simulink model "vipldwsRobot3"  (R2019a)
settings: Solver=FixedStepDiscrete  StartTime=0.0  StopTime=inf  RelTol=1e-3  EnableMultiTasking=on
model workspace (MATLAB code in the model file):
  | % Image size
  | imgSize = [240 360];
  | 
  | % Number of rows and columns in the image region to process.
  | numRows = floor(imgSize(1)/2);
  | numCols = imgSize(2);
  | 
  | % To handle different video sizes other than [240 360], scaling the Hough
  | % transform rho values by the below factor is required.
  | factor = sqrt(sum(imgSize.^2)) / sqrt(sum([240 360].^2));
  | 
  | %% parameters for the second lane
  | %approximately 35:45 (0-based index: 414:424)
  | startIdxRho_R = floor(factor * 414);
  | NumRhos_R = floor(factor * 11);
  | 
  | %approximately -90:-70 degrees (0-based index: 0:20)
  | startIdxTheta_R = 0;
  | NumThetas_R = 21;
  | neighborhood_R =  [min(7,NumRhos_R), min(7,NumThetas_R)];
  | 
  | %approximately 379:415 (0-based index: 0:35)
  | startIdxRho_L = floor(factor * 379);
  | NumRhos_L = floor(factor * 36);
  | 
  | %approximately 55:85 degrees (0-based index: 145: 175)
  | startIdxTheta_L = 145;
  | NumThetas_L = 21;
  | neighborhood_L =  [min(7,NumRhos_L), min(7,NumThetas_L)];
  | 
  | % Maximum number of lanes to find in the current frame.
  | expLaneNum = 2;
  | 
  | % Maximum number of lanes to store in the tracking repository.
  | maxLaneNum = 20;
  | 
  | % Angular resolution of Hough transform, i.e., the width of a theta bin is
  | % pi/angleNum.
  | angleNum = 180;
  | 
  | % Maximum allowable change of lane distance metric between two frames.
  | trackThreshold = 75;
  | 
  | % Minimum number of frames a lane must be detected to become a valid lane.
  | frameFound = 5;
  | 
  | % Maximum number of frames a lane can be missed without marking it invalid.
  | frameLost = 20;
  | 
  | % Size of the neighborhood around the maxima over which the Hough
  | % transforms values are suppressed. (Used in Find Local Maxima block)
  | neighborhood = [301, 81];
  | 
  | % Distance threshold for lane crossing warning; valid range is (0, 0.5).
  | thrWarn = 0.4;
  | 
  | % Weight (tweaking factor) of the angular difference for calculating the
  | % distance metric between two lanes. It is typically chosen to be close
  | % to the input image rows.
  | distanceMetricWeight = 200;
  | 
  | % Audio track used for lane cross warning.
  | load viprumbling.mat;
undefined symbols (not defined in the file or in its folder): gray, High, none, num_targets, Rec, SDTV, slselsubs, videoinput
libraries: simulink x19, visiontextngfix x8, robotlib x5, visiontransforms x4, dspmtrx3 x3, visionconversions x3, visionstatistics x3, dspsigops x2, dspindex x2, dspswit3 x2, dspstat3 x2, simulink_need_slupdate x2
(part 1 of 2)
settings Model: FPTRunName=Active  ExtModeAutoUpdateStatusClock=off  Creator=The MathWorks, Inc.  LastModifiedBy=ryoma
settings DataIOCC: LimitDataPoints=on  SaveFormat=Array  SaveOutput=off  SaveTime=off  ReturnWorkspaceOutputs=off
settings OptimizationCC: ExpressionDepthLimit=2147483647  LocalBlockOutputs=off  InitFltsAndDblsToZero=on  EfficientMapNaN2IntZero=off  LifeSpan=inf  BufferReusableBoundary=off
settings DebuggingCC: UnderspecifiedInitializationDetection=Classic  MergeDetectMultiDrivingBlocksExec=none  SignalResolutionControl=TryResolveAllWithWarning  SolverPrmCheckMsg=warning  InheritedTsInSrcMsg=none  MultiTaskDSMMsg=warning  SigSpecEnsureSampleTimeMsg=none  IntegerOverflowMsg=none  Int32ToFloatConvMsg=none  ParameterPrecisionLossMsg=none  FcnCallInpInsideContextMsg=warning  AllowSymbolicDim=off  UnknownTsInhSupMsg=none  StateNameClashWarn=warning  SFUnexpectedBacktrackingDiag=warning  SFNoUnconditionalDefaultTransitionDiag=warning  SFExecutionAtInitializationDiag=none  IntegerSaturationMsg=none  ArithmeticOperatorsInVariantConditions=warning
settings HardwareCC: ProdBitPerPointer=32  ProdBitPerSizeT=32  ProdBitPerPtrDiffT=32  ProdLargestAtomicFloat=None  ProdIntDivRoundTo=Undefined  ProdEndianess=Unspecified  ProdWordSize=32  ProdHWDeviceType=32-bit Generic  TargetBitPerPointer=64  TargetBitPerSizeT=64  TargetBitPerPtrDiffT=64  TargetLongLongMode=on  TargetIntDivRoundTo=Zero  TargetEndianess=LittleEndian  TargetWordSize=64  TargetHWDeviceType=Generic->MATLAB Host Computer  ProdEqTarget=off
settings ModelReferenceCC: PropagateSignalLabelsOutOfModel=off
settings SFSimCC: SimUseLocalCustomCode=off  SimParseCustomCode=off
settings RTWCC: RTWUseLocalCustomCode=off
settings CodeAppCC: StateflowObjectComments=on
settings GRTTargetCC: TargetFcnLib=ansi_tfl_tmw_new.mat  TargetLangStandard=C89/C90 (ANSI)  GeneratePreprocessorConditionals=Disable all  CombineOutputUpdateFcns=off  GRTInterface=on
settings ConfigComp: CovMetricSettings=dw  CovHtmlReporting=on  CovSaveCumulativeToWorkspaceVar=on  CovSaveSingleToWorkspaceVar=on  CovExternalEMLEnable=off

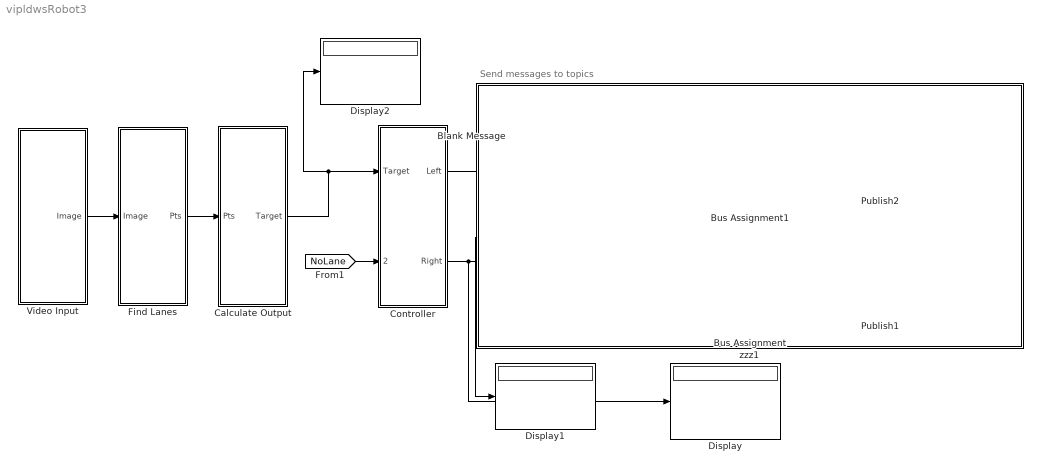
== system vipldwsRobot3 ==
  note: Send messages to topics
  Blank Message : robotlib/Blank Message  messageClass=Message  entityType=std_msgs/Int64  messageType=std_msgs/Int64  SampleTime=inf
      settings: SourceProductBaseCode=RO
  Bus Assignment : BusAssignment  AssignedSignals=Data
  Bus Assignment1 : BusAssignment  AssignedSignals=Data
  Calculate Output : Subsystem
  Controller : Subsystem
  Display : Display
  Display1 : Display
  Display2 : Display
  Find Lanes : Subsystem
  Publish1 : robotlib/Publish  topicSource=Select from ROS network  topic=/right_motor/cmd_vel  messageType=std_msgs/Int64  messageQueueLength=105
      settings: SourceProductBaseCode=RO
  Publish2 : robotlib/Publish  topicSource=Select from ROS network  topic=/left_motor/cmd_vel  messageType=std_msgs/Int64  messageQueueLength=105
      settings: SourceProductBaseCode=RO
  Video Input : Subsystem
  zzz1 : Subsystem  TreatAsAtomicUnit=on
      settings: OpenFcn=% no-op
      mask Display: disp('')
  wires:
  Video Input/1(Image) -> Find Lanes/1(Image)
  Find Lanes/1(Pts) -> Calculate Output/1(Pts)
  Bus Assignment1/1 -> Publish2/1
  Bus Assignment/1 -> Publish1/1
  Blank Message/1 -> Bus Assignment/1, Bus Assignment1/1
  Calculate Output/1(Target) -> Controller/1(Target), Display2/1
  [NoLane] -> Controller/2(No Lane)
  Controller/1(Left) -> Display1/1, Bus Assignment1/2
  Controller/2(Right) -> Bus Assignment/2, Display/1

== system vipldwsRobot3/Calculate Output ==
  Pts : Inport
  Add1 : Sum
  Constant : Constant  Value=160
  Convert 2-D to 1-D : dspsigattribs/Convert 2-D to 1-D
      settings: SourceProductName=DSP System Toolbox  SourceProductBaseCode=DS
  Demux1 : Demux  Outputs=8
  Display : Display
  Display1 : Display
  Gain : Gain  Gain=255/160
  Gain1 : Gain  Gain=.5
  Subtract : Sum  Inputs=+-
  Terminator{,1..5} (6 alike) : Terminator
  Target : Outport
  wires:
  Demux1/6 -> Add1/2, Display1/1  "right far x"
  Demux1/2 -> Display/1, Add1/1  "left far x"
  Pts/1 -> Convert 2-D to 1-D/1
  Convert 2-D to 1-D/1 -> Demux1/1
  Demux1/1 -> Terminator/1  "left far y"
  Demux1/3 -> Terminator1/1  "left close y"
  Demux1/4 -> Terminator2/1  "left close x"
  Demux1/5 -> Terminator3/1  "right far y"
  Demux1/7 -> Terminator4/1  "right close y"
  Demux1/8 -> Terminator5/1  "right close x"
  Constant/1 -> Subtract/2
  Add1/1 -> Gain1/1
  Gain1/1 -> Subtract/1
  Subtract/1 -> Gain/1
  Gain/1 -> Target/1

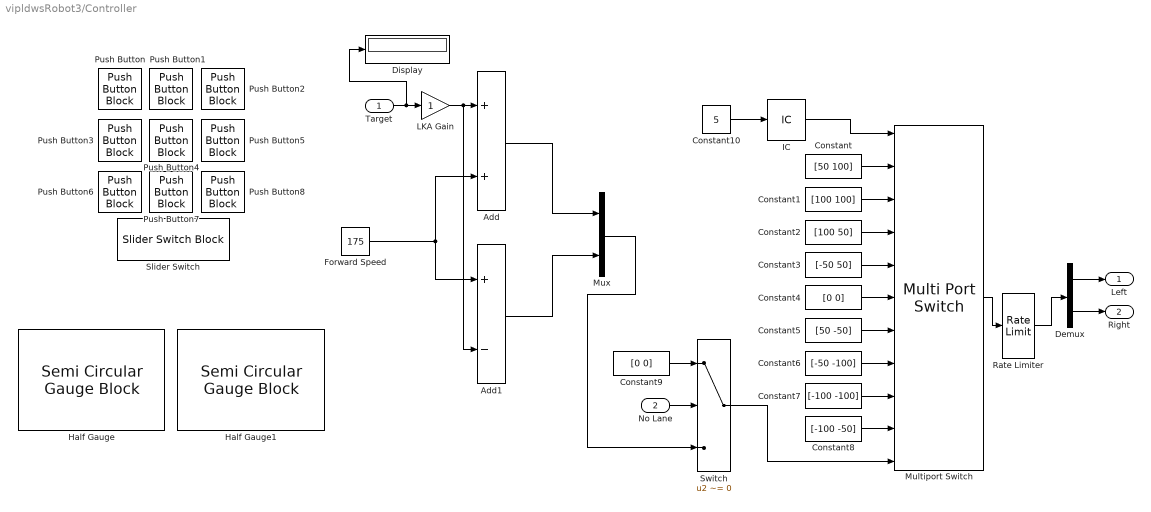
== system vipldwsRobot3/Controller ==
  Target : Inport
  No Lane : Inport  Port=2
  Add : Sum
  Add1 : Sum  Inputs=+-
  Constant : Constant  Value=[50 100]
  Constant1 : Constant  Value=[100 100]
  Constant10 : Constant  Value=5
  Constant2 : Constant  Value=[100 50]
  Constant3 : Constant  Value=[-50 50]
  Constant4 : Constant  Value=[0 0]
  Constant5 : Constant  Value=[50 -50]
  Constant6 : Constant  Value=[-50 -100]
  Constant7 : Constant  Value=[-100 -100]
  Constant8 : Constant  Value=[-100 -50]
  Constant9 : Constant  Value=[0 0]
  Demux : Demux  Outputs=2
  Display : Display
  Forward Speed : Constant  Value=175
  Half Gauge : SemiCircularGaugeBlock  ScaleMin=-255  ScaleMax=255
  Half Gauge1 : SemiCircularGaugeBlock  ScaleMin=-255  ScaleMax=255
  IC : InitialCondition  Value=5
  LKA Gain : Gain
  Multiport Switch : MultiPortSwitch  Inputs=10
  Mux : Mux  Inputs=2
  Push Button : PushButtonBlock  ButtonText=< /\
  Push Button1 : PushButtonBlock  ButtonText=/\  OnValue=2
  Push Button2 : PushButtonBlock  ButtonText=/\ >  OnValue=3
  Push Button3 : PushButtonBlock  ButtonText=<  OnValue=4
  Push Button4 : PushButtonBlock  ButtonText=0  OnValue=5
  Push Button5 : PushButtonBlock  ButtonText=>  OnValue=6
  Push Button6 : PushButtonBlock  ButtonText=< \/  OnValue=7
  Push Button7 : PushButtonBlock  ButtonText=\/  OnValue=8
  Push Button8 : PushButtonBlock  ButtonText=\/ >  OnValue=9
  Rate Limiter : RateLimiter  RisingSlewLimit=150  FallingSlewLimit=-150  SampleTimeMode=inherited
  Slider Switch : SliderSwitchBlock
      settings: Values={{'Off', 'On'}, [5 10]}
  Switch : Switch  Criteria=u2 ~= 0
  Left : Outport
  Right : Outport  Port=2
  wires:
  Forward Speed/1 -> Add1/1, Add/2
  Target/1 -> Display/1, LKA Gain/1
  LKA Gain/1 -> Add1/2, Add/1
  Add/1 -> Mux/1
  Add1/1 -> Mux/2
  No Lane/1 -> Switch/2
  Mux/1 -> Switch/3
  Rate Limiter/1 -> Demux/1
  Demux/1 -> Left/1
  Demux/2 -> Right/1
  Constant2/1 -> Multiport Switch/4
  Constant5/1 -> Multiport Switch/7
  Constant1/1 -> Multiport Switch/3
  Constant4/1 -> Multiport Switch/6
  Constant3/1 -> Multiport Switch/5
  Constant/1 -> Multiport Switch/2
  Constant7/1 -> Multiport Switch/9
  Constant8/1 -> Multiport Switch/10
  Multiport Switch/1 -> Rate Limiter/1
  Constant6/1 -> Multiport Switch/8
  Constant9/1 -> Switch/1
  Switch/1 -> Multiport Switch/11
  Constant10/1 -> IC/1
  IC/1 -> Multiport Switch/1

== system vipldwsRobot3/Find Lanes ==
  note: Lane Departure Warning System
  note: Double-click the Switch to specify
      | whether the demo highlights the lane
      | in front of the vehicle using a polygon or two lines.
  note: Copyright 2006-2011 The MathWorks, Inc.
  Image : Inport
  Departure Warning : Subsystem
  Draw Lines : Constant  Value=0  VectorParams1D=off  OutDataTypeStr=boolean
  Draw Polygon : Constant  VectorParams1D=off  OutDataTypeStr=boolean
  Info : vipmisc/Info  SystemSampleTime=-1
      settings: SourceProductName=Computer Vision Toolbox  SourceProductBaseCode=VP
  Input : Subsystem
  Lane Detection : Subsystem
  Lane Tracking : Subsystem
  Logical Operator : Logic  AllPortsSameDT=off  OutDataTypeStr=boolean
  Output : Subsystem
  Switch : ManualSwitch  CurrentSetting=0
  Pts : Outport
  wires:
  Departure Warning/4(Show3rdLane) -> Output/6(Show3rdLane)
  Input/4(YCbCrLow) -> [RefImg], Departure Warning/4(YCbCrLow)
  [R3rd] -> Output/8(R3rd)
  [RefImg] -> Output/10(RefImg)
  Draw Lines/1 -> Switch/1
  Image/1 -> Input/1("Image ")
  [L3rd] -> Output/9(L3rd)
  Input/2(EOF) -> Output/2(EOF), Lane Tracking/1(EOF)
  Input/3(ILow) -> Lane Detection/1(ILow), Departure Warning/3(ILow)
  Lane Tracking/1(Repository) -> Departure Warning/1(Repository)
  Departure Warning/6(TwoLanesFlag) -> Logical Operator/1, Output/11(TwoLanesFlag)
  Lane Detection/2(Enable) -> Lane Tracking/3(Enable)
  Departure Warning/3(Dis) -> Output/5(Dis)
  Lane Detection/1(Line) -> Lane Tracking/2(Line)
  Lane Tracking/2(Count) -> Departure Warning/2(Count)
  Departure Warning/5(ColorAndTypeIdx) -> Output/7(ColorAndTypeIdx)
  Departure Warning/1(Pts) -> Pts/1, Output/3(Pts)
  Departure Warning/2(Message) -> Output/4(Message)
  Draw Polygon/1 -> Switch/2
  Logical Operator/1 -> Output/12(ShowPolygon)
  Switch/1 -> Logical Operator/2
  Input/1(RGB) -> Output/1(RGB)
  Lane Detection/3(Right_3rdLane) -> [R3rd]
  Lane Detection/4(Left_3rdLane) -> [L3rd]

== system vipldwsRobot3/Video Input ==
  note: Receive messages sent to /usb_cam/image_raw topic
  After Blend : VideoViewer  FigPos=[46 541 418 304]
  Compositing1 : visiontextngfix/Compositing  operation=Blend  bFacSrc=Specify via dialog  bFactor=1  mFacSrc=Specify via dialog  mFactor=1  source=Specify via dialog  coordinates=[1 1]  roundingMode=Floor  overflowMode=off  firstCoeffSlope=2^-14  prodOutputMode=Binary point scaling  prodOutputWordLength=32  prodOutputFracLength=10  prodOutputSlope=2^-10  accumSlope=2^-10  outputSlope=2^-10
      settings: SourceProductName=Computer Vision Toolbox  SourceProductBaseCode=VP
  Constant : Constant  Value=[100 0 5 240; 220 0 5 240]  VectorParams1D=off  OutDataTypeStr=int32  SampleTime=1/30
  DrawShapes : visiontextngfix/Draw Shapes  shape=Rectangles  fill=on  lineWidth=1  fillClrSource=Specify via dialog  display=White  intensity=200  color=[255 255 255]  opacity=1  viewport=Entire image  antialiasing=off  inType=Obsolete  imagePorts=One multidimensional signal  roundingMode=Floor  overflowMode=off  memoryMode=Specify word length  memoryWordLength=16  prodOutputMode=Binary point scaling  prodOutputWordLength=32  prodOutputFracLength=14  prodOutputSlope=2^-14  accumSlope=2^-14  memoryFracLength=14
      settings: SourceProductName=Computer Vision Toolbox
  From Video Device : imaqlib/From Video Device  DeviceMenu=winvideo 1 (HD WebCam)  Device=winvideo 1 (HD WebCam)  ObjConstructor=videoinput('winvideo', 1)  VideoFormatMenu=MJPG_640x480  VideoFormat=MJPG_640x480  VideoSource=input1  ROIPosition=[0 0 480 640]  EnableHWTrigger=off  TriggerConfiguration=none/none  SampleTime=1/30  OutputPortsMode=One multidimensional signal  DataType=single  CanDoHWTrigger=no  ReturnedColorSpace=rgb  BlockHandle=1351.0002  ROIWidth=640  ROIHeight=480  ROIColumn=0  ROIRow=0  EngXMLPath=C:\Program Files\MATLAB\R2019a\toolbox\imaq\imaq\private  DevXMLPath=C:\ProgramData\MATLAB\SupportPackages\R2019a\toolbox\imaq\supportpackages\genericvideo\adaptor\win64  EngLibPath=C:\Program Files\MATLAB\R2019a\toolbox\imaq\imaqblks\imaqmex\win64  ColorSpace=rgb  BayerSensorAlignment=grbg  ImaqMode=off
      settings: SourceProductName=Image Acquisition Toolbox
  Image From File : visionsources/Image From File  Tag=vipblks_nd  FileName=C:\Users\ryoma\Desktop\rosmotor\windows\1x1.png  Ts=1/30  imagePorts=One multidimensional signal  OutPortLabels=R|G|B  ImageDataType=Inherit from input image  sdImageDataType=uint(8)  Signed=on  WordLength=16  FractionLengthMode=User-defined  FractionLength=15
      settings: SourceProductName=Computer Vision Toolbox
  Read Image : robotlib/Read Image  MaximumImageSize=[480, 640]  ImageEncoding=rgb8  ShowAlphaOutput=off  ShowErrorCodeOutput=off  VariableSizeOutputs=off
      settings: SourceProductName=Robotics System Toolbox  SourceProductBaseCode=RO
  Resize : visiongeotforms/Resize  specify=Output size as a percentage of input size  rfactor=50  outCols=25  outRows=25  outRowsCols=[25 35]  interp_method=Bilinear  antialias=on  useROI=off  roiFlag=off  roundingMode=Nearest  overflowMode=on  prodOutputMode=Binary point scaling  prodOutputWordLength=32  prodOutputFracLength=10  prodOutputSlope=2^-10  accumSlope=2^-10  outputSlope=2^-10
      settings: SourceProductName=Computer Vision Toolbox  SourceProductBaseCode=VP
  Resize1 : visiongeotforms/Resize  specify=Output size as a percentage of input size  rfactor=50  outCols=25  outRows=25  outRowsCols=[25 35]  interp_method=Bilinear  antialias=on  useROI=off  roiFlag=off  roundingMode=Nearest  overflowMode=on  prodOutputMode=Binary point scaling  prodOutputWordLength=32  prodOutputFracLength=10  prodOutputSlope=2^-10  accumSlope=2^-10  outputSlope=2^-10
      settings: SourceProductName=Computer Vision Toolbox  SourceProductBaseCode=VP
  Sample and Hold : dspsigops/Sample and Hold  Commented=on  trig=Rising edge  initCond=0  latchinput=off
  Step : Step  SampleTime=1/30
  Subscribe1 : robotlib/Subscribe  topicSource=Select from ROS network  topic=/usb_cam/image_raw  messageType=sensor_msgs/Image  sampleTime=1/30  messageQueueLength=51
      settings: SourceProductBaseCode=RO
  Switch : Switch  Criteria=u2 > Threshold
  zzz2 : Subsystem  TreatAsAtomicUnit=on
      settings: OpenFcn=% no-op
      mask Display: disp('')
  Image : Outport
  wires:
  From Video Device/1 -> Resize/1
  Subscribe1/2 -> Read Image/1
  Subscribe1/1 -> Sample and Hold/Trigger
  Read Image/1 -> Resize1/1
  DrawShapes/1 -> Switch/3
  Constant/1 -> DrawShapes/2
  Step/1 -> Switch/2
  Resize1/1 -> Compositing1/2
  Compositing1/1 -> DrawShapes/1, Switch/1, After Blend/1
  Image From File/1 -> Compositing1/1
  Switch/1 -> Image/1

== system vipldwsRobot3/zzz1 ==

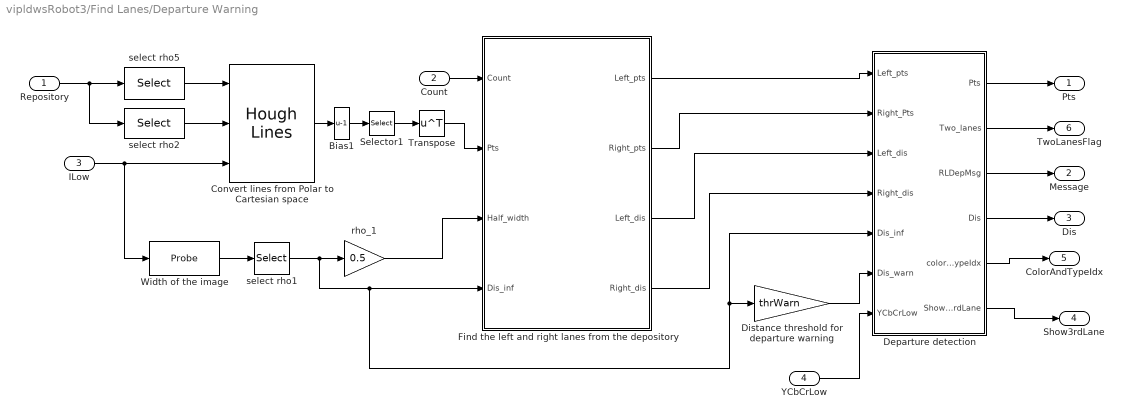
== system vipldwsRobot3/Find Lanes/Departure Warning ==
  Repository : Inport
  Count : Inport  Port=2
  ILow : Inport  Port=3
  YCbCrLow : Inport  Port=4
  Bias1 : Bias  Bias=-1
  Convert lines from Polar to Cartesian space : visiontransforms/Hough Lines  sineCompMethod=Trigonometric function  thetaRes=pi/180  roundingMode=Nearest  overflowMode=on  firstCoeffMode=Specify word length  firstCoeffWordLength=16  prodOutputMode=Binary point scaling  prodOutputWordLength=32  prodOutputFracLength=16  prodOutputSlope=2^-16  accumSlope=2^-16  firstCoeffFracLength=15
      settings: SourceProductName=Computer Vision Toolbox  SourceProductBaseCode=VP
  Departure detection : Subsystem
  Distance threshold for departure warning : Gain  Gain=thrWarn  OutDataTypeStr=Inherit: Same as input
  Find the left and right lanes from the depository : Subsystem  TreatAsAtomicUnit=on
  Selector1 : Selector  NumberOfDimensions=2  InputPortWidth=3  IndexOptions=Select all,Index vector (dialog)  Indices=[2 1],[2 1 4 3]  OutputSizes=1,1
  Transpose : Math  Operator=transpose  SaturateOnIntegerOverflow=on
  Width of the image : Probe  ProbeWidth=off  ProbeSampleTime=off  ProbeComplexSignal=off  ProbeSignalDimensions=on  ProbeDimensionsDataType=int32
  rho_1 : Gain  Gain=0.5  OutDataTypeStr=Inherit: Same as input
  select rho1 : Selector  InputPortWidth=2  IndexOptions=Index vector (dialog)  Indices=2  OutputSizes=1
  select rho2 : Selector  NumberOfDimensions=2  InputPortWidth=maxLaneNum  IndexOptions=Index vector (dialog),Select all  Indices=1,-1  OutputSizes=1
  select rho5 : Selector  NumberOfDimensions=2  InputPortWidth=maxLaneNum  IndexOptions=Index vector (dialog),Select all  Indices=2,-1  OutputSizes=1
  Pts : Outport
  Message : Outport  Port=2
  Dis : Outport  Port=3
  Show3rdLane : Outport  Port=4
  ColorAndTypeIdx : Outport  Port=5
  TwoLanesFlag : Outport  Port=6
  wires:
  select rho2/1 -> Convert lines from Polar to Cartesian space/2
  Count/1 -> Find the left and right lanes from the depository/1(Count)
  Repository/1 -> select rho5/1, select rho2/1
  ILow/1 -> Convert lines from Polar to Cartesian space/3, Width of the image/1
  select rho1/1 -> rho_1/1, Find the left and right lanes from the depository/4(Dis_inf), Distance threshold for departure warning/1, Departure detection/5(Dis_inf)
  Find the left and right lanes from the depository/2(Right_pts) -> Departure detection/2(Right_Pts)
  Find the left and right lanes from the depository/1(Left_pts) -> Departure detection/1(Left_pts)
  rho_1/1 -> Find the left and right lanes from the depository/3(Half_width)
  Width of the image/1 -> select rho1/1
  Find the left and right lanes from the depository/3(Left_dis) -> Departure detection/3(Left_dis)
  Find the left and right lanes from the depository/4(Right_dis) -> Departure detection/4(Right_dis)
  Distance threshold for departure warning/1 -> Departure detection/6(Dis_warn)
  Departure detection/1(Pts) -> Pts/1
  Departure detection/2(Two_lanes) -> TwoLanesFlag/1
  Departure detection/3(RLDepMsg) -> Message/1
  Departure detection/4(Dis) -> Dis/1
  select rho5/1 -> Convert lines from Polar to Cartesian space/1
  YCbCrLow/1 -> Departure detection/7(YCbCrLow)
  Departure detection/6(Show3rdLane) -> Show3rdLane/1
  Departure detection/5(colorAndTypeIdx) -> ColorAndTypeIdx/1
  Selector1/1 -> Transpose/1
  Convert lines from Polar to Cartesian space/1 -> Bias1/1
  Transpose/1 -> Find the left and right lanes from the depository/2(Pts)
  Bias1/1 -> Selector1/1

== system vipldwsRobot3/Find Lanes/Input ==
  note: For different video sizes, set imgSize appropriately in model
      | workspace and then press the "Reinitialize from Source" button.
  "Image " : Inport
  Clip image : dspmtrx3/Submatrix  RowSpan=Range of rows  RowStartMode=Index  RowStartIndex=numRows+1  RowEndMode=Last  RowEndIndex=1  ColSpan=All columns  ColStartMode=First  ColStartIndex=1  ColEndMode=Last  ColEndIndex=1
  Color Space Conversion : visionconversions/Color Space  Conversion  conversion=Obsolete  conversionActive=R'G'B' to intensity  wp_str=D65  rec=Rec. 601 (SDTV)  sys=1125/60/2:1  imagePorts=One multidimensional signal
  Color Space Conversion1 : visionconversions/Color Space  Conversion  conversion=Obsolete  conversionActive=R'G'B' to Y'CbCr  wp_str=D65  rec=Rec. 601 (SDTV)  sys=1125/60/2:1  imagePorts=One multidimensional signal
  From Multimedia File1 : dspvision/From Multimedia File  Commented=on  inputFilename=viplanedeparture.mp4  readRange=[1 Inf]  loop=on  numPlays=inf  outputStreams=Video only  videoDataType=single  audioDataType=int16  inheritSampleTime=off  userDefinedSampleTime=1/30  noAudioOutput=off  isIntensityVideo=off  fourcc=RGB  colorVideoFormat=One multidimensional signal  outputEOF=on  dataOrg=Column-major  audioFrameSize=1024  computeAudioFrameSize=off  outSamplingMode=Frame based
      settings: SourceProductName=DSP System Toolbox  SourceProductBaseCode=DS
  OR : Logic  Operator=OR  IconShape=distinctive  AllPortsSameDT=off  OutDataTypeStr=boolean
  Selector : Selector  NumberOfDimensions=3  InputPortWidth=3  IndexOptions=Index vector (dialog),Select all,Select all  Indices=(numRows+1):imgSize(1),1,2  OutputSizes=1,1,1
  RGB : Outport
  EOF : Outport  Port=2
  ILow : Outport  Port=3
  YCbCrLow : Outport  Port=4
  tag scope: NoLane=global
  wires:
  Color Space Conversion/1 -> Clip image/1
  Clip image/1 -> ILow/1
  Selector/1 -> Color Space Conversion1/1
  Color Space Conversion1/1 -> YCbCrLow/1
  "Image "/1 -> Selector/1, Color Space Conversion/1, RGB/1
  [Lane0R] -> OR/2
  [Lane0L] -> OR/1
  OR/1 -> EOF/1, [NoLane]

== system vipldwsRobot3/Find Lanes/Lane Detection ==
  ILow : Inport
  2-D FIR Filter : visionfilter/2-D FIR Filter  separable=off  filtSrc=Specify via dialog  filterMtrx=[-1 0 1]  verticalFilter=[4 0]  horizontalFilter=[4 0]  outSize=Same as input port I  padType=Replicate  padSrc=Specify via dialog  padVal=0  method=Correlation  firstCoeffMode=Specify word length  firstCoeffWordLength=16  firstCoeffFracLength=14  firstCoeffSignedness=Signed  firstCoeffLastDataTypeStr=fixdt(1,16)  outputSignedness=Auto  accumLastDataTypeStr=Inherit: Same as product output  prodOutputMode=Binary point scaling  prodOutputWordLength=32  prodOutputFracLength=10  prodOutputLastDataTypeStr=fixdt([],32,10)  roundingMode=Floor  overflowMode=on  firstCoeffDataTypeStr=fixdt(1,16)  firstCoeffMin=[]  firstCoeffMax=[]  prodOutputDataTypeStr=fixdt([],32,10)  accumDataTypeStr=Inherit: Same as product output  outputMin=[]  outputMax=[]
      settings: SourceProductName=Computer Vision Toolbox  SourceProductBaseCode=VP
  3rd lane: Right-Left : Subsystem
  Hough Transform : visiontransforms/Hough Transform  theta_res=pi/angleNum  rho_res=1  out_theta_rho=on  outdtmode=single  roundingMode=Nearest  overflowMode=on  firstCoeffMode=Binary point scaling  firstCoeffWordLength=16  firstCoeffFracLength=14  firstCoeffSlope=2^-14  secondCoeffMode=Binary point scaling  secondCoeffWordLength=32  secondCoeffFracLength=16  secondCoeffSlope=2^-16  prodOutputMode=Binary point scaling  prodOutputWordLength=32  prodOutputFracLength=20  prodOutputSlope=2^-20  accumMode=Binary point scaling  accumWordLength=32  accumFracLength=20  accumSlope=2^-20  outputMode=Binary point scaling  outputWordLength=16  outputFracLength=0  outputSlope=2^0  memoryMode=Binary point scaling  memoryWordLength=32  memoryFracLength=16  memorySlope=2^-16
      settings: SourceProductName=Computer Vision Toolbox  SourceProductBaseCode=VP
  Image thresholding : visionconversions/Autothreshold  operator=>  threshOut=off  effMetricOut=off  userDefinedRange=off  umin=0  umax=255  outOfRngOpt=Warn and saturate  scaleThreshold=off  scaleFactor=1  roundingMode=Floor  overflowMode=off  P1Mode=Specify word length  P1WordLength=32  P1FracLength=30  P1Slope=2^-30  A1Slope=2^-30  P2Mode=Specify word length  P2WordLength=32  P2FracLength=22  P2Slope=2^-22  A2Slope=2^-22  P3Mode=Specify word length  P3WordLength=32  P3FracLength=14  P3Slope=2^-14  A3Slope=2^-14  P4Mode=Binary point scaling  P4WordLength=32  P4FracLength=15  P4Slope=2^-15  A4Slope=2^-4  Q1Mode=Specify word length  Q1WordLength=32  Q1FracLength=16  Q1Slope=2^-16  EMMode=Specify word length  EMWordLength=16  EMFracLength=14  EMSlope=2^-14
      settings: SourceProductName=Computer Vision Toolbox  SourceProductBaseCode=VP
  Overwrite : Subsystem
  Peak detection : Subsystem
  Saturation : Saturate  UpperLimit=1  LowerLimit=0
  Line : Outport
  Enable : Outport  Port=2
  Right_3rdLane : Outport  Port=3
  Left_3rdLane : Outport  Port=4
  wires:
  Overwrite/1(Out) -> Peak detection/1(Hough)
  3rd lane: Right-Left/2(LeftPts) -> Left_3rdLane/1
  3rd lane: Right-Left/1(RightPts) -> Right_3rdLane/1
  Peak detection/2(Enable) -> Enable/1
  Peak detection/1(Line) -> Line/1
  Hough Transform/3 -> Peak detection/3(Rho_list), 3rd lane: Right-Left/3(rho_list)
  Hough Transform/2 -> Peak detection/2(Theta_list), 3rd lane: Right-Left/2(th_list)
  Hough Transform/1 -> Overwrite/1(In), 3rd lane: Right-Left/1(H)
  Saturation/1 -> Image thresholding/1
  2-D FIR Filter/1 -> Saturation/1
  Image thresholding/1 -> Hough Transform/1
  ILow/1 -> 2-D FIR Filter/1, 3rd lane: Right-Left/4(Ref I)

== system vipldwsRobot3/Find Lanes/Lane Tracking ==
  EOF : Inport
  Line : Inport  Port=2
  Enable : Inport  Port=3
  Kalman Filter : dspadpt3/Kalman Filter  num_targets=maxLaneNum  sourceEnable=Specify via input port <Enable>  isReset=on  X=zeros([4, 1])  P=100*eye(4)  A=[1 0 1 0;0 1 0 1; 0 0 1 0; 0 0 0 1]  sourceMeasure=Specify via Dialog  H=[1 0 0 0; 0 1 0 0]  Q=0.05*eye(4)  R=1*eye(2)  isOutputEstMeasure=on  isOutputEstState=off  isOutputEstError=off  isOutputPrdMeasure=on  isOutputPrdState=off  isOutputPrdError=off
      settings: SourceProductName=DSP System Toolbox  SourceProductBaseCode=DS
  Matching : Subsystem
  Only update the lines which Kalman filter has been trained for enough time : simulink/Logic and Bit Operations/Compare To Constant  relop=>=  const=frameFound  OutDataTypeStr=boolean  ZeroCross=off
  Unit Delay Resettable : simulink_need_slupdate/Unit Delay Resettable  vinit=0  tsamp=-1
      settings: SourceProductName=Simulink  SourceProductBaseCode=SL
  Unit Delay Resettable1 : simulink_need_slupdate/Unit Delay Resettable  vinit=zeros(2,maxLaneNum)  tsamp=-1
      settings: SourceProductName=Simulink  SourceProductBaseCode=SL
  Update : Subsystem  TreatAsAtomicUnit=on
  Repository : Outport
  Count : Outport  Port=2
  wires:
  Matching/2(Count) -> Unit Delay Resettable/1, Only update the lines which Kalman filter has been trained for enough time/1, Count/1, Kalman Filter/2
  Only update the lines which Kalman filter has been trained for enough time/1 -> Update/3(Update)
  Unit Delay Resettable/1 -> Matching/4(Count_ref)
  Unit Delay Resettable1/1 -> Matching/3(Rep_ref)
  Line/1 -> Matching/1(Line)
  Enable/1 -> Matching/2(Enable)
  Matching/1(Repository) -> Update/1(Old), Kalman Filter/1
  Update/1(Out) -> Unit Delay Resettable1/1
  Kalman Filter/2 -> Update/2(New)
  Kalman Filter/1 -> Repository/1
  EOF/1 -> Unit Delay Resettable1/2, Unit Delay Resettable/2

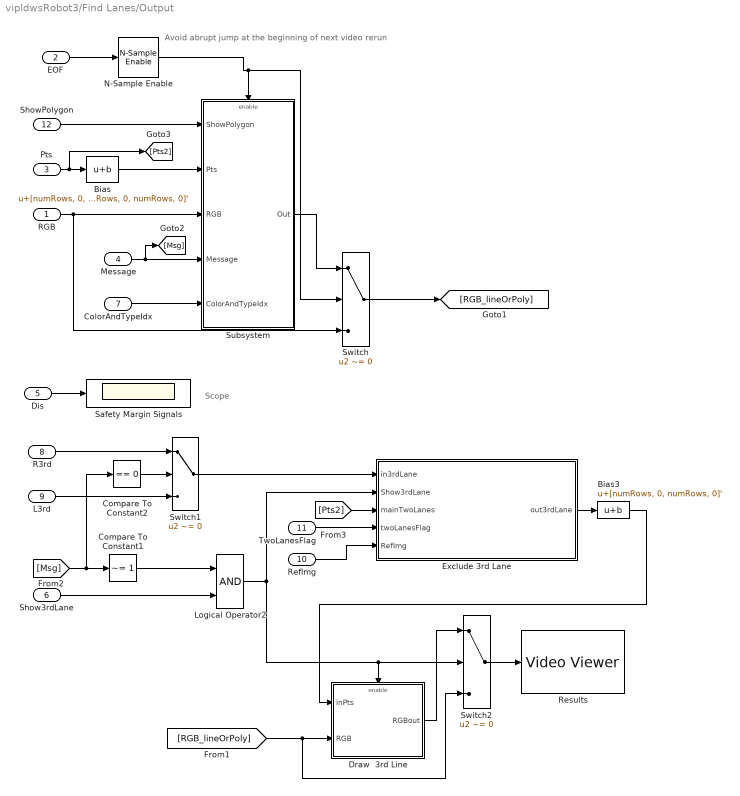
== system vipldwsRobot3/Find Lanes/Output ==
  note: Scope
  note: Avoid abrupt jump at the beginning of next video rerun
  RGB : Inport
  EOF : Inport  Port=2
  Pts : Inport  Port=3
  Message : Inport  Port=4
  Dis : Inport  Port=5
  Show3rdLane : Inport  Port=6
  ColorAndTypeIdx : Inport  Port=7
  R3rd : Inport  Port=8
  L3rd : Inport  Port=9
  RefImg : Inport  Port=10
  TwoLanesFlag : Inport  Port=11
  ShowPolygon : Inport  Port=12
  Bias : Bias  Bias=[numRows, 0, numRows, 0; numRows, 0, numRows, 0]'
  Bias3 : Bias  Bias=[numRows, 0, numRows, 0]'
  Compare To Constant1 : simulink/Logic and Bit Operations/Compare To Constant  relop=~=  const=1  OutDataTypeStr=boolean  ZeroCross=off
  Compare To Constant2 : simulink/Logic and Bit Operations/Compare To Constant  relop===  const=0  OutDataTypeStr=boolean  ZeroCross=off
  Draw  3rd Line : Subsystem  TreatAsAtomicUnit=on
  Exclude 3rd Lane : MATLAB Function  TreatAsAtomicUnit=on
  Logical Operator2 : Logic  AllPortsSameDT=off  OutDataTypeStr=boolean
  N-Sample Enable : dspswit3/N-Sample Enable  N=8  ActiveLevel=High (1)  reset=on  TriggerType=Non-zero sample  Ts=1  DataType=Logical
      settings: SourceProductName=DSP System Toolbox  SourceProductBaseCode=DS
  Results : VideoViewer  colormapValue=gray(256)  FigPos=[842 424 491 266]
  Safety Margin Signals : Scope
  Subsystem : Subsystem
  Switch : Switch  Criteria=u2 ~= 0
  Switch1 : Switch  Criteria=u2 ~= 0  ZeroCross=off
  Switch2 : Switch  Criteria=u2 ~= 0
  wires:
  Pts/1 -> Bias/1, [Pts2]
  Message/1 -> Subsystem/4(Message), [Msg]
  Dis/1 -> Safety Margin Signals/1
  Bias/1 -> Subsystem/2(Pts)
  ColorAndTypeIdx/1 -> Subsystem/5(ColorAndTypeIdx)
  Show3rdLane/1 -> Logical Operator2/2
  [RGB_lineOrPoly] -> Draw  3rd Line/2(RGB), Switch2/3
  [Msg] -> Compare To Constant1/1, Compare To Constant2/1
  Compare To Constant1/1 -> Logical Operator2/1
  Logical Operator2/1 -> Exclude 3rd Lane/2(Show3rdLane), Draw  3rd Line/Enable, Switch2/2
  Compare To Constant2/1 -> Switch1/2
  Switch1/1 -> Exclude 3rd Lane/1(in3rdLane)
  Draw  3rd Line/1(RGBout) -> Switch2/1
  Switch2/1 -> Results/1
  [Pts2] -> Exclude 3rd Lane/3(mainTwoLanes)
  TwoLanesFlag/1 -> Exclude 3rd Lane/4(twoLanesFlag)
  RefImg/1 -> Exclude 3rd Lane/5(RefImg)
  Exclude 3rd Lane/1(out3rdLane) -> Bias3/1
  R3rd/1 -> Switch1/1
  L3rd/1 -> Switch1/3
  ShowPolygon/1 -> Subsystem/1(ShowPolygon)
  RGB/1 -> Subsystem/3(RGB), Switch/3
  N-Sample Enable/1 -> Switch/2, Subsystem/Enable
  EOF/1 -> N-Sample Enable/1
  Bias3/1 -> Draw  3rd Line/1(inPts)
  Switch/1 -> [RGB_lineOrPoly]
  Subsystem/1(Out) -> Switch/1

== system vipldwsRobot3/Video Input/zzz2 ==

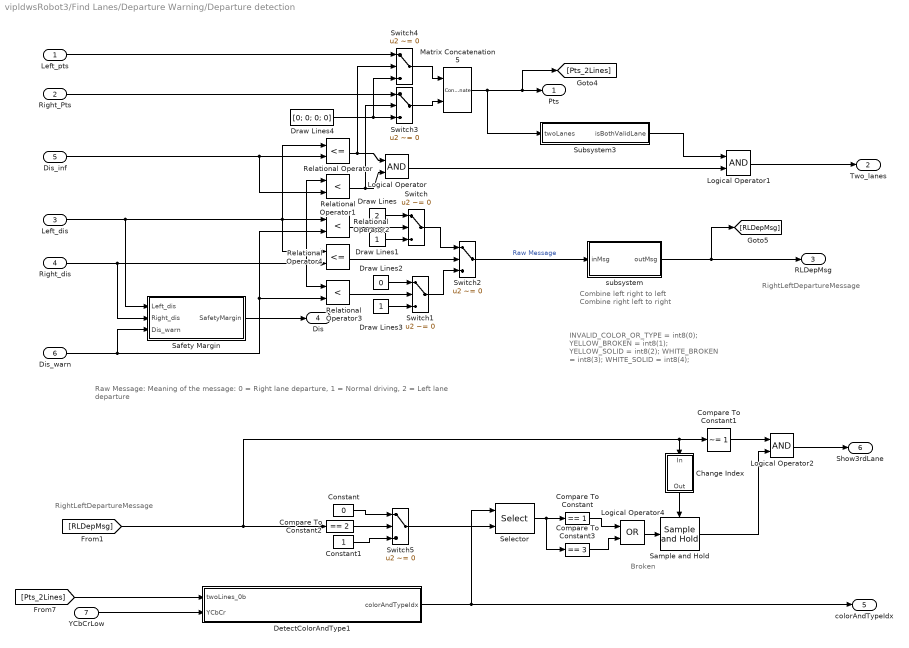
== system vipldwsRobot3/Find Lanes/Departure Warning/Departure detection ==
  note: Raw Message:
      | Meaning of the message: 0 = Right lane departure, 1 = Normal driving, 2 = Left lane departure
  note: RightLeftDepartureMessage
  note: INVALID_COLOR_OR_TYPE = int8(0);
      | YELLOW_BROKEN  = int8(1);
      | YELLOW_SOLID      = int8(2);
      | WHITE_BROKEN     = int8(3);
      | WHITE_SOLID         = int8(4);
  note: Broken
  note: RightLeftDepartureMessage
  note: Combine left right to left
      | Combine right left to right
  Left_pts : Inport
  Right_Pts : Inport  Port=2
  Left_dis : Inport  Port=3
  Right_dis : Inport  Port=4
  Dis_inf : Inport  Port=5
  Dis_warn : Inport  Port=6
  YCbCrLow : Inport  Port=7
  Change Index : Subsystem
  Compare To Constant : simulink/Logic and Bit Operations/Compare To Constant  relop===  const=1  OutDataTypeStr=boolean  ZeroCross=off
  Compare To Constant1 : simulink/Logic and Bit Operations/Compare To Constant  relop=~=  const=1  OutDataTypeStr=boolean  ZeroCross=off
  Compare To Constant2 : simulink/Logic and Bit Operations/Compare To Constant  relop===  const=2  OutDataTypeStr=boolean  ZeroCross=off
  Compare To Constant3 : simulink/Logic and Bit Operations/Compare To Constant  relop===  const=3  OutDataTypeStr=boolean  ZeroCross=off
  Constant : Constant  Value=0  VectorParams1D=off  OutDataTypeStr=int8
  Constant1 : Constant  VectorParams1D=off  OutDataTypeStr=int8
  DetectColorAndType1 : MATLAB Function  TreatAsAtomicUnit=on
  Draw Lines : Constant  Value=2  VectorParams1D=off  OutDataTypeStr=int8  SampleTime=-1
  Draw Lines1 : Constant  VectorParams1D=off  OutDataTypeStr=int8  SampleTime=-1
  Draw Lines2 : Constant  Value=0  VectorParams1D=off  OutDataTypeStr=int8  SampleTime=-1
  Draw Lines3 : Constant  VectorParams1D=off  OutDataTypeStr=int8  SampleTime=-1
  Draw Lines4 : Constant  Value=[0; 0; 0; 0]  VectorParams1D=off  OutDataTypeStr=int32  SampleTime=-1
  Logical Operator : Logic  AllPortsSameDT=off  OutDataTypeStr=boolean
  Logical Operator1 : Logic  AllPortsSameDT=off  OutDataTypeStr=boolean
  Logical Operator2 : Logic  AllPortsSameDT=off  OutDataTypeStr=boolean
  Logical Operator4 : Logic  Operator=OR  AllPortsSameDT=off  OutDataTypeStr=boolean
  Matrix Concatenation5 : Concatenate  Mode=Multidimensional array  ConcatenateDimension=2
  Relational Operator : RelationalOperator  Operator=<=  OutDataTypeStr=boolean  ZeroCross=off  RndMeth=Nearest
  Relational Operator1 : RelationalOperator  Operator=<  OutDataTypeStr=boolean  ZeroCross=off  RndMeth=Nearest
  Relational Operator2 : RelationalOperator  Operator=<  OutDataTypeStr=boolean  ZeroCross=off  RndMeth=Nearest
  Relational Operator3 : RelationalOperator  Operator=<  OutDataTypeStr=boolean  ZeroCross=off  RndMeth=Nearest
  Relational Operator4 : RelationalOperator  Operator=<=  OutDataTypeStr=boolean  ZeroCross=off  RndMeth=Nearest
  Safety Margin : Subsystem
  Sample and Hold : dspsigops/Sample and Hold  trig=Either edge  initCond=0  latchinput=off
  Selector : Selector  IndexMode=Zero-based  InputPortWidth=2  IndexOptions=Index vector (port)  Indices=[1 3]  OutputSizes=1
  Subsystem3 : Subsystem
  Switch : Switch  Criteria=u2 ~= 0
  Switch1 : Switch  Criteria=u2 ~= 0
  Switch2 : Switch  Criteria=u2 ~= 0
  Switch3 : Switch  Criteria=u2 ~= 0  ZeroCross=off
  Switch4 : Switch  Criteria=u2 ~= 0  ZeroCross=off
  Switch5 : Switch  Criteria=u2 ~= 0  ZeroCross=off
  subsystem : Subsystem
  Pts : Outport
  Two_lanes : Outport  Port=2
  RLDepMsg : Outport  Port=3
  Dis : Outport  Port=4
  colorAndTypeIdx : Outport  Port=5
  Show3rdLane : Outport  Port=6
  wires:
  Relational Operator1/1 -> Logical Operator/2, Switch3/2
  Relational Operator/1 -> Logical Operator/1, Switch4/2
  Switch1/1 -> Switch2/3
  Switch/1 -> Switch2/1
  Relational Operator4/1 -> Switch2/2
  Draw Lines3/1 -> Switch1/3
  Draw Lines2/1 -> Switch1/1
  Draw Lines1/1 -> Switch/3
  Draw Lines/1 -> Switch/1
  Relational Operator3/1 -> Switch1/2
  Relational Operator2/1 -> Switch/2
  Dis_warn/1 -> Relational Operator2/2, Relational Operator3/2, Safety Margin/3(Dis_warn)
  Left_dis/1 -> Relational Operator2/1, Relational Operator4/1, Relational Operator/1, Safety Margin/1(Left_dis)
  Right_dis/1 -> Relational Operator1/1, Relational Operator4/2, Relational Operator3/1, Safety Margin/2(Right_dis)
  Dis_inf/1 -> Relational Operator/2, Relational Operator1/2
  Switch3/1 -> Matrix Concatenation5/2
  Switch4/1 -> Matrix Concatenation5/1
  Draw Lines4/1 -> Switch3/3, Switch4/3
  Left_pts/1 -> Switch4/1
  Matrix Concatenation5/1 -> Subsystem3/1(twoLanes), Pts/1, [Pts_2Lines]
  Right_Pts/1 -> Switch3/1
  Switch2/1 -> subsystem/1(inMsg)  "Raw Message"
  subsystem/1(outMsg) -> RLDepMsg/1, [RLDepMsg]
  Subsystem3/1(isBothValidLane) -> Logical Operator1/1
  Logical Operator/1 -> Logical Operator1/2
  Logical Operator1/1 -> Two_lanes/1
  YCbCrLow/1 -> DetectColorAndType1/2(YCbCr)
  DetectColorAndType1/1(colorAndTypeIdx) -> colorAndTypeIdx/1, Selector/1
  Compare To Constant1/1 -> Logical Operator2/1
  Selector/1 -> Compare To Constant3/1, Compare To Constant/1
  Compare To Constant2/1 -> Switch5/2
  Switch5/1 -> Selector/2
  Compare To Constant/1 -> Logical Operator4/1
  Compare To Constant3/1 -> Logical Operator4/2
  Logical Operator4/1 -> Sample and Hold/1
  Sample and Hold/1 -> Logical Operator2/2
  Change Index/1(Out) -> Sample and Hold/Trigger
  Logical Operator2/1 -> Show3rdLane/1
  [RLDepMsg] -> Compare To Constant1/1, Change Index/1(In), Compare To Constant2/1
  Constant1/1 -> Switch5/3
  Constant/1 -> Switch5/1
  Safety Margin/1(SafetyMargin) -> Dis/1
  [Pts_2Lines] -> DetectColorAndType1/1(twoLines_0b)

== system vipldwsRobot3/Find Lanes/Departure Warning/Find the left and right lanes from the depository ==
  note: Left and right lanes are identified by their intersection positions with the bottom image boundary.
      | The intersection point of the left lane is to the left of the image bottom boundary center,
      | and is the one closest to the center. By the same way, but to the right, the right lane is defined.
  Count : Inport
  Pts : Inport  Port=2
  Half_width : Inport  Port=3
  Dis_inf : Inport  Port=4
  Compare To Constant2 : simulink/Logic and Bit Operations/Compare To Constant  relop=>=  const=frameFound  OutDataTypeStr=boolean  ZeroCross=off
  For Iterator : ForIterator  ResetStates=reset  IterationLimit=maxLaneNum
  Search for the left and right lanes : Subsystem
  select rho1 : Selector  NumberOfDimensions=2  InputPortWidth=maxLaneNum  IndexOptions=Select all,Index vector (port)  Indices=-1,-1  OutputSizes=1
  select rho5 : Selector  NumberOfDimensions=2  InputPortWidth=maxLaneNum  IndexOptions=Select all,Index vector (port)  Indices=-1,-1  OutputSizes=1
  Left_pts : Outport
  Right_pts : Outport  Port=2
  Left_dis : Outport  Port=3
  Right_dis : Outport  Port=4
  wires:
  Pts/1 -> select rho5/1
  select rho1/1 -> Compare To Constant2/1
  Half_width/1 -> Search for the left and right lanes/3(Half_width)
  select rho5/1 -> Search for the left and right lanes/2(Pts)
  Compare To Constant2/1 -> Search for the left and right lanes/1(Enable)
  Search for the left and right lanes/1(Left_pts) -> Left_pts/1
  Search for the left and right lanes/2(Left_dis) -> Left_dis/1
  Search for the left and right lanes/3(Right_pts) -> Right_pts/1
  Search for the left and right lanes/4(Right_dis) -> Right_dis/1
  For Iterator/1 -> select rho5/2, select rho1/2
  Count/1 -> select rho1/1
  Dis_inf/1 -> Search for the left and right lanes/4(Dis_inf)

== system vipldwsRobot3/Find Lanes/Lane Detection/3rd lane: Right-Left ==
  H : Inport
  th_list : Inport  Port=2
  rho_list : Inport  Port=3
  Ref I : Inport  Port=4
  Find Left 3rd Lane : Subsystem
  Find Right 3rd Lane : Subsystem
  Hough Lines : visiontransforms/Hough Lines  sineCompMethod=Trigonometric function  thetaRes=pi/180  roundingMode=Nearest  overflowMode=on  firstCoeffMode=Specify word length  firstCoeffWordLength=16  prodOutputMode=Binary point scaling  prodOutputWordLength=32  prodOutputFracLength=16  prodOutputSlope=2^-16  accumSlope=2^-16  firstCoeffFracLength=15
      settings: SourceProductName=Computer Vision Toolbox  SourceProductBaseCode=VP
  Hough Lines1 : visiontransforms/Hough Lines  sineCompMethod=Trigonometric function  thetaRes=pi/180  roundingMode=Nearest  overflowMode=on  firstCoeffMode=Specify word length  firstCoeffWordLength=16  prodOutputMode=Binary point scaling  prodOutputWordLength=32  prodOutputFracLength=16  prodOutputSlope=2^-16  accumSlope=2^-16  firstCoeffFracLength=15
      settings: SourceProductName=Computer Vision Toolbox  SourceProductBaseCode=VP
  Selector1 : Selector  NumberOfDimensions=2  InputPortWidth=3  IndexOptions=Select all,Index vector (dialog)  Indices=[2 1],[2 1 4 3]  OutputSizes=1,1
  Selector2 : Selector  NumberOfDimensions=2  InputPortWidth=3  IndexOptions=Select all,Index vector (dialog)  Indices=[2 1],[2 1 4 3]  OutputSizes=1,1
  Transpose : Math  Operator=transpose  SaturateOnIntegerOverflow=on
  Transpose1 : Math  Operator=transpose  SaturateOnIntegerOverflow=on
  RightPts : Outport
  LeftPts : Outport  Port=2
  wires:
  Ref I/1 -> Hough Lines1/3, Hough Lines/3
  Find Left 3rd Lane/2(Rho) -> Hough Lines1/2
  Find Left 3rd Lane/1(Theta) -> Hough Lines1/1
  Find Right 3rd Lane/2(Rho) -> Hough Lines/2
  Find Right 3rd Lane/1(Theta) -> Hough Lines/1
  H/1 -> Find Right 3rd Lane/1(H), Find Left 3rd Lane/1(H)
  th_list/1 -> Find Right 3rd Lane/2(th_list), Find Left 3rd Lane/2(th_list)
  rho_list/1 -> Find Right 3rd Lane/3(rho_list), Find Left 3rd Lane/3(rho_list)
  Selector1/1 -> Transpose/1
  Selector2/1 -> Transpose1/1
  Hough Lines/1 -> Selector1/1
  Transpose/1 -> RightPts/1
  Hough Lines1/1 -> Selector2/1
  Transpose1/1 -> LeftPts/1

== system vipldwsRobot3/Find Lanes/Lane Detection/Overwrite ==
  note: Wipe out Hamtrix with
      | theta >=  78deg
  note: Wipe out Hamtrix with
      | theta <  -78deg
  In : Inport
  Overwrite Values : dspmtrx3/Overwrite Values  OverWriteDiag=Submatrix  valFrom2ndIP=Specify via dialog  ConstValue=0  RowSpan=All rows  RowStartMode=First  RowStartIndex=1  RowEndMode=Last  RowEndIndex=1  ColSpan=Range of columns  ColStartMode=First  ColStartIndex=1  ColEndMode=Index  ColEndIndex=12  DiagSpan=Range of elements  DiagStartMode=Index  DiagStartIndex=2  DiagEndMode=Index  DiagEndIndex=4
      settings: SourceProductName=DSP System Toolbox  SourceProductBaseCode=DS
  Overwrite Values1 : dspmtrx3/Overwrite Values  OverWriteDiag=Submatrix  valFrom2ndIP=Specify via dialog  ConstValue=0  RowSpan=All rows  RowStartMode=First  RowStartIndex=1  RowEndMode=Last  RowEndIndex=1  ColSpan=Range of columns  ColStartMode=Offset from last  ColStartIndex=12  ColEndMode=Last  ColEndIndex=15  DiagSpan=Range of elements  DiagStartMode=Index  DiagStartIndex=2  DiagEndMode=Index  DiagEndIndex=4
      settings: SourceProductName=DSP System Toolbox  SourceProductBaseCode=DS
  Out : Outport
  wires:
  Overwrite Values/1 -> Overwrite Values1/1
  In/1 -> Overwrite Values/1
  Overwrite Values1/1 -> Out/1

== system vipldwsRobot3/Find Lanes/Lane Detection/Peak detection ==
  note: Detect lines in the image by finding the peaks in the Hough transform matrix
  Hough : Inport
  Theta_list : Inport  Port=2
  Rho_list : Inport  Port=3
  Enable signal generator : Subsystem  TreatAsAtomicUnit=on
  Find Local Maxima : visionstatistics/Find Local Maxima  num_peaks=expLaneNum  nhood_size=neighborhood  src_thresh=Obsolete9b  src_thresh_inuse=Specify via dialog  threshold=1  inputIsHough=on  dt_peak=uint16  isOutVarDim=on  dt_count=uint16
      settings: SourceProductName=Computer Vision Toolbox  SourceProductBaseCode=VP
  Matrix Concatenation3 : Concatenate  Mode=Multidimensional array
  Probe : Probe  ProbeWidth=off  ProbeSampleTime=off  ProbeComplexSignal=off  ProbeSignalDimensions=on
  Selector : Selector  NumberOfDimensions=2  InputPortWidth=3  IndexOptions=Index vector (dialog),Index vector (dialog)  Indices=1,2  OutputSizes=1,1
  Selector rho : Selector  NumberOfDimensions=2  InputPortWidth=3  IndexOptions=Select all,Index vector (port)  Indices=1,2  OutputSizes=1,1
  Selector theta : Selector  NumberOfDimensions=2  InputPortWidth=3  IndexOptions=Select all,Index vector (port)  Indices=1,2  OutputSizes=1,1
  Selector1 : Selector  NumberOfDimensions=2  InputPortWidth=3  IndexOptions=Select all,Index vector (dialog)  Indices=[2 1],[2 1]  OutputSizes=1,1
  Transpose : Math  Operator=transpose  SaturateOnIntegerOverflow=on
  Zero-Order Hold1 : ZeroOrderHold  SampleTime=-1
  Zero-Order Hold2 : ZeroOrderHold  SampleTime=-1
  select rho : Selector  NumberOfDimensions=2  InputPortWidth=3  IndexOptions=Index vector (dialog),Select all  Indices=1,-1  OutputSizes=1
  select rho3 : Selector  NumberOfDimensions=2  InputPortWidth=3  IndexOptions=Index vector (dialog),Select all  Indices=2,-1  OutputSizes=1
  Line : Outport
  Enable : Outport  Port=2
  wires:
  Hough/1 -> Find Local Maxima/1
  Enable signal generator/1(Enable) -> Enable/1
  Matrix Concatenation3/1 -> Line/1
  Selector theta/1 -> Matrix Concatenation3/2
  Selector rho/1 -> Matrix Concatenation3/1
  Zero-Order Hold1/1 -> Selector theta/1
  select rho3/1 -> Selector theta/2
  Theta_list/1 -> Zero-Order Hold1/1
  Zero-Order Hold2/1 -> Selector rho/1
  select rho/1 -> Selector rho/2
  Rho_list/1 -> Zero-Order Hold2/1
  Probe/1 -> Selector/1
  Selector/1 -> Enable signal generator/1(Num)
  Find Local Maxima/1 -> Selector1/1
  Selector1/1 -> Transpose/1
  Transpose/1 -> select rho/1, select rho3/1, Probe/1

== system vipldwsRobot3/Find Lanes/Lane Tracking/Matching ==
  Line : Inport
  Enable : Inport  Port=2
  Rep_ref : Inport  Port=3
  Count_ref : Inport  Port=4
  Calculate the distances between the lines found in the current frame and those in the repository : Subsystem  TreatAsAtomicUnit=on
  Find the best matches between the current lines and those in the repository : Subsystem  TreatAsAtomicUnit=on
  Update the repository : Subsystem  TreatAsAtomicUnit=on
  Repository : Outport
  Count : Outport  Port=2
  wires:
  Find the best matches between the current lines and those in the repository/2(Match_dis) -> Update the repository/4(Match_dis)
  Calculate the distances between the lines found in the current frame and those in the repository/1(Dis) -> Find the best matches between the current lines and those in the repository/1(Dis)
  Enable/1 -> Calculate the distances between the lines found in the current frame and those in the repository/4(Enable)
  Rep_ref/1 -> Calculate the distances between the lines found in the current frame and those in the repository/2(Rep_ref), Update the repository/1(Rep_ref)
  Line/1 -> Update the repository/5(Line), Calculate the distances between the lines found in the current frame and those in the repository/3(Line)
  Find the best matches between the current lines and those in the repository/1(Match_list) -> Update the repository/3(Match_list)
  Update the repository/1(Repository) -> Repository/1
  Update the repository/2(Count) -> Count/1
  Count_ref/1 -> Update the repository/2(Count_ref), Calculate the distances between the lines found in the current frame and those in the repository/1(Count)

== system vipldwsRobot3/Find Lanes/Lane Tracking/Update ==
  note: For each element (column), Out equals to New if Enable is true; or equals to Old otherwise.
  Old : Inport
  New : Inport  Port=2
  Update : Inport  Port=3
  Assignment : Assignment  NumberOfDimensions=2  IndexOptions=Assign all,Index vector (port)  Indices=-1,-1  OutputSizes=1,1
  For Iterator : ForIterator  ResetStates=reset  IterationLimit=maxLaneNum
  Selector : Selector  InputPortWidth=maxLaneNum  IndexOptions=Index vector (port)  Indices=[1 3]  OutputSizes=1
  Selector1 : Selector  NumberOfDimensions=2  InputPortWidth=maxLaneNum  IndexOptions=Select all,Index vector (port)  Indices=-1,1  OutputSizes=1
  Selector2 : Selector  NumberOfDimensions=2  InputPortWidth=maxLaneNum  IndexOptions=Select all,Index vector (port)  Indices=-1,1  OutputSizes=1
  Switch1 : Switch  Criteria=u2 ~= 0
  Out : Outport
  wires:
  Switch1/1 -> Assignment/2
  Selector/1 -> Switch1/2
  Selector2/1 -> Switch1/3
  Selector1/1 -> Switch1/1
  New/1 -> Assignment/1, Selector1/1
  Old/1 -> Selector2/1
  Assignment/1 -> Out/1
  Update/1 -> Selector/1
  For Iterator/1 -> Assignment/3, Selector1/2, Selector2/2, Selector/2

== system vipldwsRobot3/Find Lanes/Output/Draw  3rd Line ==
  inPts : Inport
  RGB : Inport  Port=2
  Enable : EnablePort  PropagateVarSize=During execution
  DrawShapes : visiontextngfix/Draw Shapes  shape=Lines  fill=on  lineWidth=1  fillClrSource=Specify via dialog  display=User-specified value  intensity=200  color=[0 1 0]'  opacity=0.6  viewport=Entire image  antialiasing=on  inType=Obsolete  imagePorts=One multidimensional signal  roundingMode=Floor  overflowMode=off  memoryMode=Specify word length  memoryWordLength=16  prodOutputMode=Binary point scaling  prodOutputWordLength=32  prodOutputFracLength=14  prodOutputSlope=2^-14  accumSlope=2^-14  memoryFracLength=15
      settings: SourceProductName=Computer Vision Toolbox
  Selector2 : Selector  InputPortWidth=4  IndexOptions=Index vector (dialog)  Indices=[2 1 4 3]  OutputSizes=1
  RGBout : Outport
  wires:
  DrawShapes/1 -> RGBout/1
  RGB/1 -> DrawShapes/1
  inPts/1 -> Selector2/1
  Selector2/1 -> DrawShapes/2

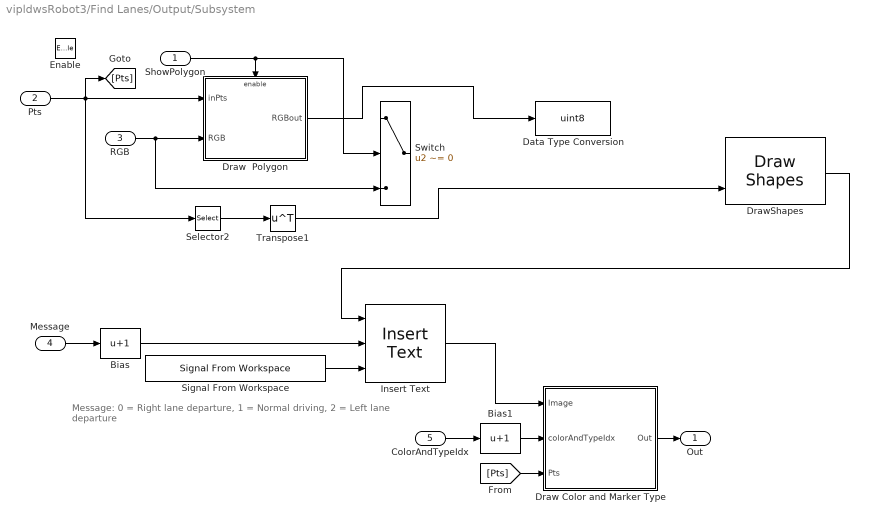
== system vipldwsRobot3/Find Lanes/Output/Subsystem ==
  note: Message:
      | 0 = Right lane departure, 1 = Normal driving, 2 = Left lane departure
  ShowPolygon : Inport
  Pts : Inport  Port=2
  RGB : Inport  Port=3
  Message : Inport  Port=4
  ColorAndTypeIdx : Inport  Port=5
  Enable : EnablePort  PropagateVarSize=During execution
  Bias : Bias  Bias=1
  Bias1 : Bias  Bias=1
  Data Type Conversion : DataTypeConversion  OutDataTypeStr=uint8
  Draw  Polygon : Subsystem  TreatAsAtomicUnit=on
  Draw Color and Marker Type : Subsystem
  DrawShapes : visiontextngfix/Draw Shapes  shape=Lines  fill=on  lineWidth=1  fillClrSource=Specify via dialog  display=User-specified value  intensity=200  color=[1 1 0; 1 0 1]  opacity=0.6  viewport=Entire image  antialiasing=on  inType=Obsolete  imagePorts=One multidimensional signal  roundingMode=Floor  overflowMode=off  memoryMode=Specify word length  memoryWordLength=16  prodOutputMode=Binary point scaling  prodOutputWordLength=32  prodOutputFracLength=14  prodOutputSlope=2^-14  accumSlope=2^-14  memoryFracLength=14
      settings: SourceProductName=Computer Vision Toolbox
  Insert Text : visiontextngfix/Insert Text  inputType=Obsolete  theText="{sprintf('                    Right\\n                    Departure'),'',sprintf(' Left\\n Departure')}"  getTextLocFrom=Specify via dialog  textLoc=[2 170]  getTextColorFrom=Input port  textColor=[1 1 1]  getTextIntensityFrom=Specify via dialog  textIntensity=0  getTextOpacityFrom=Specify via dialog  textOpacity=1  dummyVar2=0  dummyVar3=0  dummyVar4=0  imagePorts=One multidimensional signal  isInputTransposed=off  fontFace=LucidaTypewriterBold  dummyVar1=0  blockFontSize=20  antiAliased=on
      settings: SourceProductName=Computer Vision Toolbox  SourceProductBaseCode=VP
  Selector2 : Selector  NumberOfDimensions=2  InputPortWidth=3  IndexOptions=Index vector (dialog),Select all  Indices=[2 1 4 3],1  OutputSizes=1,1
  Signal From Workspace : dspsrcs4/Signal From Workspace  X=single([1 0 0;1 0 0; 0 0 0;0 0 0])  Ts=1/30  nsamps=1  OutputAfterFinalValue=Cyclic repetition  ignoreOrWarnInputAndFrameLengths=off  OutputFrames=on
  Switch : Switch  Criteria=u2 ~= 0
  Transpose1 : Math  Operator=transpose  SaturateOnIntegerOverflow=on
  Out : Outport
  wires:
  DrawShapes/1 -> Insert Text/1
  Draw  Polygon/1(RGBout) -> Data Type Conversion/1
  Signal From Workspace/1 -> Insert Text/3
  ShowPolygon/1 -> Switch/2, Draw  Polygon/Enable
  RGB/1 -> Draw  Polygon/2(RGB), Switch/3
  Insert Text/1 -> Draw Color and Marker Type/1(Image)
  Pts/1 -> Selector2/1, Draw  Polygon/1(inPts), [Pts]
  Message/1 -> Bias/1
  ColorAndTypeIdx/1 -> Bias1/1
  Draw Color and Marker Type/1(Out) -> Out/1
  [Pts] -> Draw Color and Marker Type/3(Pts)
  Selector2/1 -> Transpose1/1
  Transpose1/1 -> DrawShapes/2
  Bias/1 -> Insert Text/2
  Bias1/1 -> Draw Color and Marker Type/2(colorAndTypeIdx)

== system vipldwsRobot3/Find Lanes/Departure Warning/Departure detection/Change Index ==
  In : Inport
  Constant : Constant  Value=[0 -1 1]  VectorParams1D=off  OutDataTypeStr=int32
  Data Type Conversion : DataTypeConversion  OutDataTypeStr=int32  SaturateOnIntegerOverflow=on  RndMeth=Zero
  Selector : Selector  IndexMode=Zero-based  InputPortWidth=3  IndexOptions=Index vector (port)  Indices=[1 3]  OutputSizes=1
  Out : Outport
  wires:
  In/1 -> Data Type Conversion/1
  Selector/1 -> Out/1
  Data Type Conversion/1 -> Selector/2
  Constant/1 -> Selector/1
